simulink model "SerialSystem"  (R2014a)
settings: Solver=ode3  StartTime=0.0  StopTime=800  FixedStep=0.01  RelTol=1e-3
libraries: simulink x4
settings Model: SimulationMode=accelerator  Creator=nw010080  LastModifiedBy=nm010080
settings DebuggingCC: UnderspecifiedInitializationDetection=Classic  StateNameClashWarn=warning

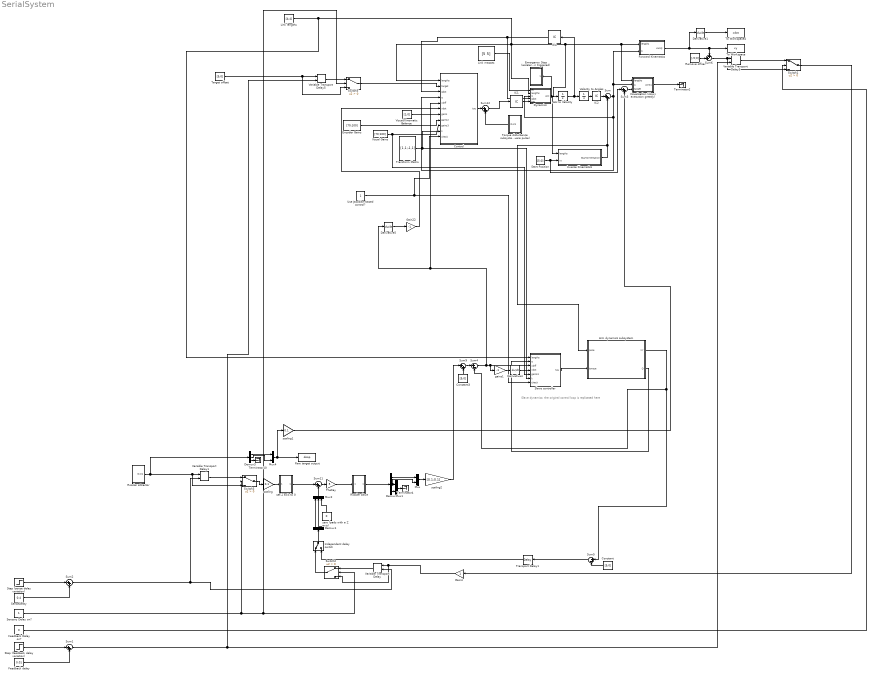
== system SerialSystem ==
  note: Slave dynamics: the original control
      | loop is replicated here
  Acc to Velocity : Integrator
  Arm dynamics subsystem : Subsystem
  Constant : Constant  Value=[5;0]
  Constant3 : Constant  Value=[5;0]
  Control : MATLAB Function  TreatAsAtomicUnit=on
  Demux : Demux  Outputs=3
  Demux1 : Demux  Outputs=2
  Demux3 : Demux  Outputs=3
  Derivative1 : Derivative
  Derivative4 : Derivative
  Derivative5 : Derivative
  Dynamics : MATLAB Function  TreatAsAtomicUnit=on
  Emergency Stop (acceleration triggered) : Subsystem
  Encoder Gains : Constant  Value=[70;100]
  Feedback Delay on? : Constant  Value=0
  Feedback delay : Constant  Value=0.01
  Forward Kinematics : MATLAB Function  TreatAsAtomicUnit=on
  Gain22 : Gain  Gain=-1
  Gain4 : Gain
  IC1 : InitialCondition  Value=[0;0]
  IC2 : InitialCondition  Value=[0;0]
  IC3 : InitialCondition  Value=[0;0]
  Independent delay switch : ManualSwitch
  Inverse Kinematics : MATLAB Function  TreatAsAtomicUnit=on
  Link lengths : Constant  Value=[4;4]
  Link masses : Constant  Value=[5 5]
  Mux : Mux  Inputs=2
  Mux1 : Mux  Inputs=2
  Mux2 : Mux  Inputs=3
  Mux4 : Mux  Inputs=2
  Raw target output : ToWorkspace  VariableName=doop  SaveFormat=Timeseries  SampleTime=-1
  Remove offset : Constant  Value=[-5;0]
  Rossler attractor : Subsystem
  Rossler slave : Subsystem
  SenseDelay : Constant  Value=0.4
  Sensory Delay on? : Constant
  Slave controller : MATLAB Function  TreatAsAtomicUnit=on
  Start Position : Constant  Value=[5;0]
  Step (feedback delay variation) : Step  Time=200  After=0.4  SampleTime=0
  Step (sense delay variation) : Step  Time=200  After=0.4  SampleTime=0
  Sum{,1..3,9,12} (6 alike) : Sum  Inputs=|++
  Sum11 : Sum  Inputs=|+-
  Sum4 : Sum  Inputs=|+-
  Sum5 : Sum  Inputs=|+-
  Sum6 : Sum  Inputs=++|
  Switch{1..3,5} (4 alike) : Switch  Criteria=u2 > Threshold
  Target offset : Constant  Value=[5;0]
  Terminator10 : Terminator
  Terminator2 : Terminator
  Terminator4 : Terminator
  TheKay : Gain  Gain=5
  To Workspace : ToWorkspace  VariableName=xy  SaveFormat=Timeseries  SampleTime=-1
  To Workspace4 : ToWorkspace  VariableName=xdot  SaveFormat=Timeseries  SampleTime=-1
  Torque disturbance subsystem (produces a single square pulse) : Subsystem
  Transform Matrix : Constant  Value=[1,1;-1,1]
  Transport Delay1 : TransportDelay  DelayTime=0.4
  Use Jacobian-based control? : Constant
  Variable Transport Delay : VariableTransportDelay  VariableDelayType=Variable transport delay  MaximumDelay=7  MaximumPoints=8024
  Variable Transport Delay1 : VariableTransportDelay  VariableDelayType=Variable transport delay  MaximumDelay=7  MaximumPoints=8024  FixedBuffer=on
  Variable Transport Delay3 : VariableTransportDelay  VariableDelayType=Variable transport delay  MaximumDelay=7  MaximumPoints=8024
  Variable Transport Delay5 : VariableTransportDelay  VariableDelayType=Variable transport delay  MaximumDelay=7  MaximumPoints=8024
  Velocity to Angles : Integrator
  Visual Gains : Constant  Value=[70;100]
  Visual/Kinematic Balance : Constant  Value=[1;0]
  Visualisation (slows execution greatly) : MATLAB Function  TreatAsAtomicUnit=on
  gains1 : Gain  Gain=-1
  scaling : Gain  Gain=0.1
  scaling1 : Gain  Gain=0.1
  scaling2 : Gain  Gain=[0.1;0.1]
  set Z axis to 0 : Subsystem
  zero (pads with a Z axis) : Constant  Value=0
  wires:
  Link lengths/1 -> Slave controller/1(lengths), Dynamics/2(lengths), Control/1(lengths), Visualisation (slows execution greatly)/1(lengths), Forward Kinematics/1(lengths), Inverse Kinematics/1(lengths)
  Visual/Kinematic Balance/1 -> Control/7(gains)
  Velocity to Angles/1 -> IC2/1
  IC2/1 -> Sum/1
  Start Position/1 -> Sum3/1, Inverse Kinematics/2(xy)
  IC3/1 -> Control/3(qdot), Dynamics/4(qdot)
  Encoder Gains/1 -> Control/8(gains2)
  Link masses/1 -> Dynamics/1(m)
  Visualisation (slows execution greatly)/1(joint1) -> Terminator2/1
  IC1/1 -> Dynamics/5(tau)
  Target offset/1 -> Switch5/3, Variable Transport Delay5/1
  Acc to Velocity/1 -> IC3/1, Velocity to Angles/1
  Derivative5/1 -> Gain22/1
  Inverse Kinematics/1(StartOrientation) -> Arm dynamics subsystem/1(pose), Sum/2
  Visual Gains/1 -> Slave controller/5(gains3), Control/9(gains3)
  gains1/1 -> Derivative4/1
  Derivative4/1 -> Slave controller/4(xdot)
  Gain22/1 -> Control/6(xdot)
  Constant3/1 -> Sum9/2
  Sum9/1 -> Sum4/1
  Sum11/1 -> TheKay/1
  Mux2/1 -> Sum11/2
  scaling/1 -> set Z axis to 0/1(In1)
  Demux/2 -> Mux/2, Mux1/1
  Demux/3 -> Mux1/2
  Mux1/1 -> Terminator4/1
  Demux/1 -> Mux/1
  zero (pads with a Z axis)/1 -> Mux2/3
  Demux1/2 -> Mux2/2
  Sum1/1 -> Variable Transport Delay5/2, Variable Transport Delay3/2
  Sum12/1 -> IC1/1
  Dynamics/1(acc) -> Acc to Velocity/1, Emergency Stop (acceleration triggered)/1(Acceleration)
  Demux1/1 -> Mux2/1
  Sum2/1 -> Variable Transport Delay/2, Variable Transport Delay1/2
  SenseDelay/1 -> Sum2/2
  Step (sense delay variation)/1 -> Sum2/1
  Sum3/1 -> Visualisation (slows execution greatly)/3(target)
  scaling2/1 -> Sum9/1
  TheKay/1 -> Rossler slave/1(In1)
  Mux/1 -> scaling2/1
  Transform Matrix/1 -> Control/10(k), Slave controller/6(k)
  Derivative1/1 -> To Workspace4/1
  set Z axis to 0/1(Out1) -> Sum11/1
  Switch5/1 -> Control/2(target)
  Feedback Delay on?/1 -> Switch1/2
  Switch3/1 -> scaling/1
  Switch1/1 -> Gain4/1
  Demux3/3 -> Terminator10/1
  Rossler slave/1(Out1) -> Demux/1
  Arm dynamics subsystem/2(Q) -> Slave controller/2(q)
  Variable Transport Delay1/1 -> Switch3/1
  Mux4/1 -> scaling1/1, Raw target output/1
  Demux3/2 -> Mux4/2
  Demux3/1 -> Mux4/1
  Sum/1 -> Control/4(q), Dynamics/3(q), Forward Kinematics/2(q), Visualisation (slows execution greatly)/2(q)
  Gain4/1 -> Variable Transport Delay/1, Switch2/3
  Remove offset/1 -> Sum6/2
  Sum6/1 -> Switch1/3, Variable Transport Delay3/1
  Slave controller/1(tau) -> Arm dynamics subsystem/2(torque)
  Arm dynamics subsystem/1(XY) -> Sum5/1, Sum4/2
  Sum4/1 -> gains1/1, Slave controller/3(xdiff), Derivative5/1, Control/5(xdiff)
  Rossler attractor/1(Out1) -> Switch3/3, Variable Transport Delay1/1, Demux3/1
  Control/1(tau) -> Sum12/1
  Variable Transport Delay3/1 -> Switch1/1
  Use Jacobian-based control?/1 -> Control/11(check), Slave controller/7(check)
  Sensory Delay on?/1 -> Switch5/2, Switch2/2, Switch3/2
  Variable Transport Delay/1 -> Switch2/1
  Variable Transport Delay5/1 -> Switch5/1
  Forward Kinematics/1(xandy) -> To Workspace/1, Sum6/1, Derivative1/1
  Sum5/1 -> Transport Delay1/1
  Constant/1 -> Sum5/2
  Transport Delay1/1 -> Independent delay switch/2
  Switch2/1 -> Independent delay switch/1
  Independent delay switch/1 -> Demux1/1
  Torque disturbance subsystem (produces a single square pulse)/1(Out1) -> Sum12/2
  Step (feedback delay variation)/1 -> Sum1/1
  Feedback delay/1 -> Sum1/2
  scaling1/1 -> Sum3/2

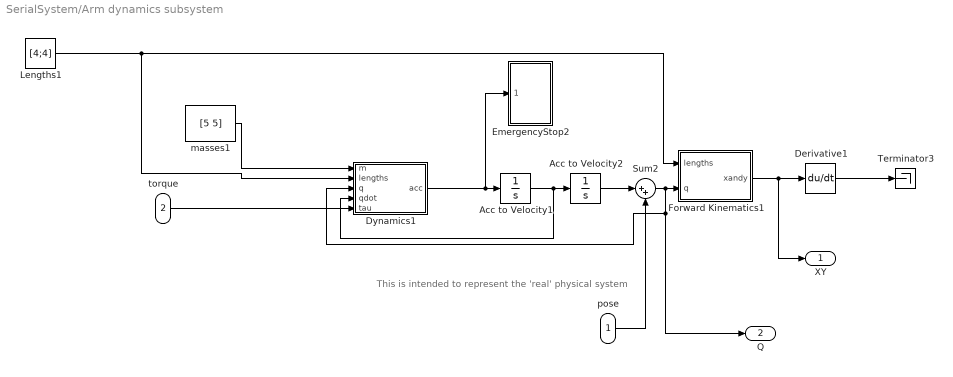
== system SerialSystem/Arm dynamics subsystem ==
  note: This is intended to represent the 'real' physical system
  pose : Inport
  torque : Inport  Port=2
  Acc to Velocity1 : Integrator
  Acc to Velocity2 : Integrator
  Derivative1 : Derivative
  Dynamics1 : MATLAB Function  TreatAsAtomicUnit=on
  EmergencyStop2 : Subsystem
  Forward Kinematics1 : MATLAB Function  TreatAsAtomicUnit=on
  Lengths1 : Constant  Value=[4;4]
  Sum2 : Sum  Inputs=|++
  Terminator3 : Terminator
  masses1 : Constant  Value=[5 5]
  XY : Outport
  Q : Outport  Port=2
  wires:
  torque/1 -> Dynamics1/5(tau)
  Forward Kinematics1/1(xandy) -> XY/1, Derivative1/1
  Acc to Velocity2/1 -> Sum2/1
  Lengths1/1 -> Dynamics1/2(lengths), Forward Kinematics1/1(lengths)
  Sum2/1 -> Q/1, Dynamics1/3(q), Forward Kinematics1/2(q)
  masses1/1 -> Dynamics1/1(m)
  Derivative1/1 -> Terminator3/1
  pose/1 -> Sum2/2
  Acc to Velocity1/1 -> Dynamics1/4(qdot), Acc to Velocity2/1
  Dynamics1/1(acc) -> EmergencyStop2/1(Acceleration), Acc to Velocity1/1

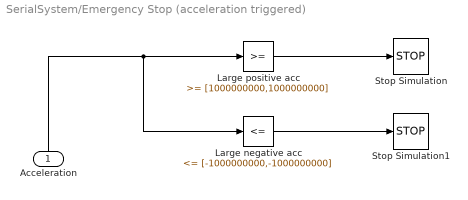
== system SerialSystem/Emergency Stop (acceleration triggered) ==
  Acceleration : Inport
  Large negative acc : simulink/Logic and Bit Operations/Compare To Constant  relop=<=  const=[-1000000000,-1000000000]  OutDataTypeStr=boolean
  Large positive acc : simulink/Logic and Bit Operations/Compare To Constant  relop=>=  const=[1000000000,1000000000]  OutDataTypeStr=boolean
  Stop Simulation : Stop
  Stop Simulation1 : Stop
  wires:
  Large negative acc/1 -> Stop Simulation1/1
  Large positive acc/1 -> Stop Simulation/1
  Acceleration/1 -> Large negative acc/1, Large positive acc/1

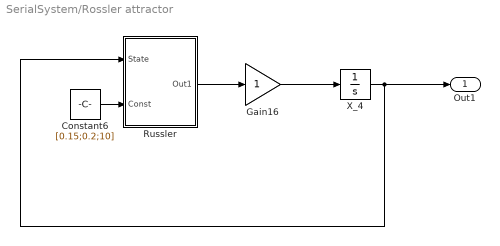
== system SerialSystem/Rossler attractor ==
  Constant6 : Constant  Value=[0.15;0.2;10]
  Gain16 : Gain
  Russler : Subsystem
  X_4 : Integrator  InitialCondition=[-1;1;0]*0
  Out1 : Outport
  wires:
  X_4/1 -> Russler/1(State), Out1/1
  Gain16/1 -> X_4/1
  Russler/1(Out1) -> Gain16/1
  Constant6/1 -> Russler/2(Const)

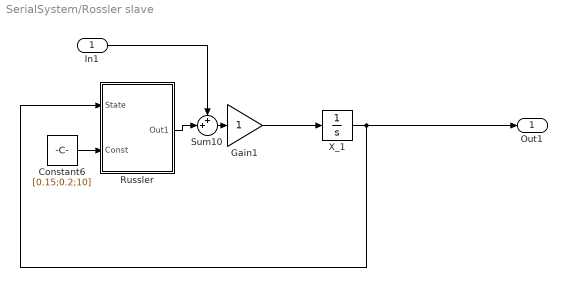
== system SerialSystem/Rossler slave ==
  In1 : Inport
  Constant6 : Constant  Value=[0.15;0.2;10]
  Gain1 : Gain
  Russler : Subsystem
  Sum10 : Sum  Inputs=++|
  X_1 : Integrator  InitialCondition=[0;0;0]
  Out1 : Outport
  wires:
  Constant6/1 -> Russler/2(Const)
  In1/1 -> Sum10/1
  Sum10/1 -> Gain1/1
  Russler/1(Out1) -> Sum10/2
  Gain1/1 -> X_1/1
  X_1/1 -> Out1/1, Russler/1(State)

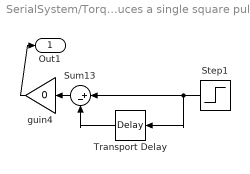
== system SerialSystem/Torque disturbance subsystem (produces a single square pulse) ==
  Step1 : Step  Time=300  SampleTime=0
  Sum13 : Sum  Inputs=|+-
  Transport Delay : TransportDelay  DelayTime=0.2
  guin4 : Gain  Gain=0
  Out1 : Outport
  wires:
  Step1/1 -> Sum13/1, Transport Delay/1
  Transport Delay/1 -> Sum13/2
  guin4/1 -> Out1/1
  Sum13/1 -> guin4/1

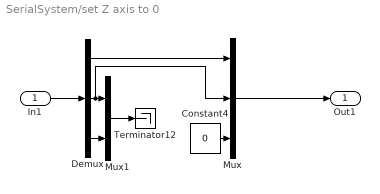
== system SerialSystem/set Z axis to 0 ==
  In1 : Inport
  Constant4 : Constant  Value=0
  Demux : Demux  Outputs=3
  Mux : Mux  Inputs=3
  Mux1 : Mux  Inputs=2
  Terminator12 : Terminator
  Out1 : Outport
  wires:
  Demux/1 -> Mux/1
  In1/1 -> Demux/1
  Mux1/1 -> Terminator12/1
  Demux/3 -> Mux1/2
  Demux/2 -> Mux/2, Mux1/1
  Constant4/1 -> Mux/3
  Mux/1 -> Out1/1

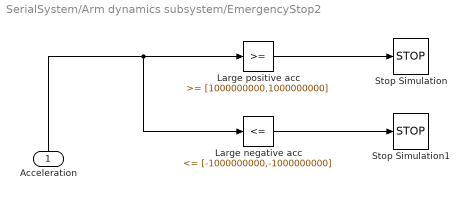
== system SerialSystem/Arm dynamics subsystem/EmergencyStop2 ==
  Acceleration : Inport
  Large negative acc : simulink/Logic and Bit Operations/Compare To Constant  relop=<=  const=[-1000000000,-1000000000]  OutDataTypeStr=boolean
  Large positive acc : simulink/Logic and Bit Operations/Compare To Constant  relop=>=  const=[1000000000,1000000000]  OutDataTypeStr=boolean
  Stop Simulation : Stop
  Stop Simulation1 : Stop
  wires:
  Large negative acc/1 -> Stop Simulation1/1
  Large positive acc/1 -> Stop Simulation/1
  Acceleration/1 -> Large negative acc/1, Large positive acc/1

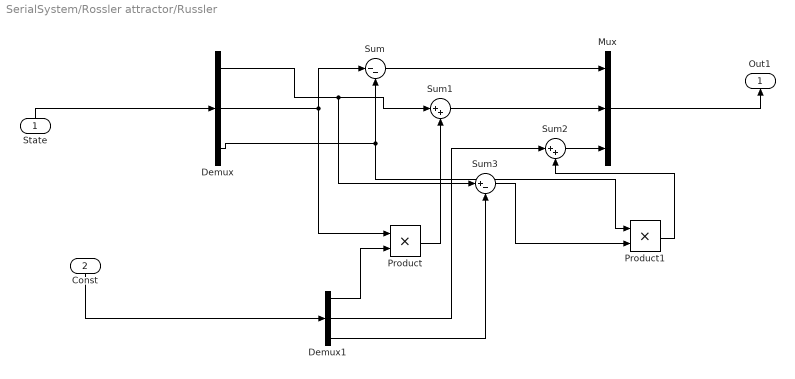
== system SerialSystem/Rossler attractor/Russler ==
  State : Inport
  Const : Inport  Port=2
  Demux : Demux  Outputs=3
  Demux1 : Demux  Outputs=3
  Mux : Mux  Inputs=3
  Product : Product
  Product1 : Product
  Sum : Sum  Inputs=|--
  Sum1 : Sum  Inputs=|++
  Sum2 : Sum  Inputs=|++
  Sum3 : Sum  Inputs=|+-
  Out1 : Outport
  wires:
  Demux1/2 -> Sum2/1
  Sum3/1 -> Product1/2
  Const/1 -> Demux1/1
  Demux/1 -> Sum3/1, Sum1/1
  Demux/2 -> Sum/1, Product/1
  Product1/1 -> Sum2/2
  Demux1/3 -> Sum3/2
  Sum/1 -> Mux/1
  Sum2/1 -> Mux/3
  Product/1 -> Sum1/2
  Mux/1 -> Out1/1
  Demux1/1 -> Product/2
  Sum1/1 -> Mux/2
  State/1 -> Demux/1
  Demux/3 -> Product1/1, Sum/2

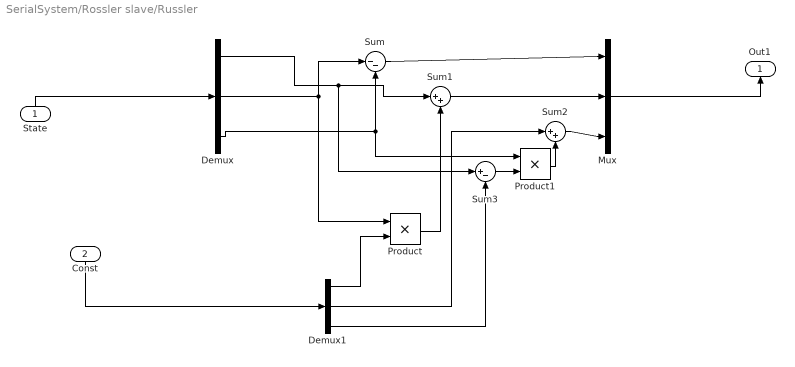
== system SerialSystem/Rossler slave/Russler ==
  State : Inport
  Const : Inport  Port=2
  Demux : Demux  Outputs=3
  Demux1 : Demux  Outputs=3
  Mux : Mux  Inputs=3
  Product : Product
  Product1 : Product
  Sum : Sum  Inputs=|--
  Sum1 : Sum  Inputs=|++
  Sum2 : Sum  Inputs=|++
  Sum3 : Sum  Inputs=|+-
  Out1 : Outport
  wires:
  Demux/3 -> Sum/2, Product1/1
  State/1 -> Demux/1
  Sum1/1 -> Mux/2
  Demux1/1 -> Product/2
  Mux/1 -> Out1/1
  Product/1 -> Sum1/2
  Sum2/1 -> Mux/3
  Sum/1 -> Mux/1
  Demux1/3 -> Sum3/2
  Product1/1 -> Sum2/2
  Demux/2 -> Product/1, Sum/1
  Demux/1 -> Sum1/1, Sum3/1
  Const/1 -> Demux1/1
  Sum3/1 -> Product1/2
  Demux1/2 -> Sum2/1

== matlab function SerialSystem/Forward Kinematics ==
  data: lengths input; xandy output; q input
function xandy  = fKinematics(lengths, q)
% forward kinematics equations
l1 = lengths(1);
l2 = lengths(2);

x = l1*cos(q(1)) + l2*cos(q(1)+q(2));
y = l1*sin(q(1)) + l2*sin(q(1)+q(2));

xandy = [x;y];

== matlab function SerialSystem/Control ==
  data: lengths input; tau output; target input; qdot input; q input; xdiff input; xdot input; gains input; gains2 input; gains3 input; k input; check input
function tau  = control(lengths, target, qdot, q, xdiff, xdot, gains,gains2, gains3, k, check)
queue = q;% get joint positions
l1 = lengths(1);
l2 = lengths(2);

if(target(1)^2 + target(2)^2 > (l1+l2-0.02)^2)% caps target to within arm reach, preventing ensuring the inverse kinematics return a real solution
    targ1 = target(1)*((l1+l2-0.02)/sqrt(target(1)^2+target(2)^2));
    targ2 = target(2)*((l1+l2-0.02)/sqrt(target(1)^2+target(2)^2));
    target = [targ1;targ2];
end

% extract gain values
m1 = gains(1);
m2 = gains(2);
kp = gains3(1);
kv = gains3(2);
gp = gains2(1);
gv = gains2(2);


% place into diagonal gain matrices
tau = [0;0];

M1 = [m1,0;0,m1];%camera gain
M2 = [m2,0;0,m2];%encoder gain

Kp = [kp,0;0,kp];% 'camera' position feedback gain
kv = [kv,0;0,kv];% 'camera' velocity feedback gain

Gp = [gp,0;0,gp];% jointspace position feedback gain
Gv = [gv,0;0,gv];% jointspace velocity feedback gain

%---------------------------------Inverse kinematics-----------------------
d1 = (target(1)^2 + target(2)^2 + l1^2 - l2^2)/(2*l1);
d2 = (target(1)^2 + target(2)^2 - l1^2 + l2^2)/(2*l2);

Q1 = atan2(target(2),target(1)) - atan2(sqrt(target(1)^2 + target(2)^2 - d1^2),d1);
Q2 = atan2(sqrt(target(1)^2 + target(2)^2 - d1^2),d1) + atan2(sqrt(target(1)^2 + target(2)^2 - d2^2),d2);
%--------------------------------------------------------------------------

desiredq = [Q1;Q2];% target joint angles

J=[-l1*sin(q(1))-l2*sin(q(1)+q(2)), -l2*sin(q(1)+q(2)); l1*cos(q(1))+l2*cos(q(1)+q(2)), l2*cos(q(1)+q(2))];% Robot arm Jacobian
if(check)
    k = J';% transpose Jacobian for force control
end

cam = M1*(Kp*k*(xdiff)-kv*k*xdot);% visual feedback terms
internal = M2*(Gp*(desiredq-queue)-Gv*qdot);%kinematic feedback terms

% true = [-l1*sin(q(1))-l2*sin(q(1)+q(2)), -l2*sin(q(1)+q(2)); l1*cos(q(1))+l2*cos(q(1)+q(2)), l2*cos(q(1)+q(2))]'*xdot;
% est = k*xdot;

tau = cam + internal;% calculate total torque

== matlab function SerialSystem/Inverse Kinematics ==
  data: lengths input; StartOrientation output; xy input
function StartOrientation  = iKinematics(lengths, xy)
l1 = lengths(1);
l2 = lengths(2);

StartOrientation = zeros(2,1);

d1 = (xy(1)^2 + xy(2)^2 + l1^2 - l2^2)/(2*l1);
d2 = (xy(1)^2 + xy(2)^2 - l1^2 + l2^2)/(2*l2);

StartOrientation(1) = atan2(xy(2),xy(1)) - atan2(sqrt(xy(1)^2 + xy(2)^2 - d1^2),d1);
StartOrientation(2) = atan2(sqrt(xy(1)^2 + xy(2)^2 - d1^2),d1) + atan2(sqrt(xy(1)^2 + xy(2)^2 - d2^2),d2);

== matlab function SerialSystem/Visualisation (slows execution greatly) ==
  data: lengths input; q input; target input; joint1 output
function joint1 = vis(lengths, q, target)
l1 = lengths(1);
l2 = lengths(2);

jointx = [0, l1*cos(q(1)), l1*cos(q(1))+l2*cos(q(1)+q(2))];% x positions of arm joints and end effector
jointy = [0, l1*sin(q(1)), l1*sin(q(1))+l2*sin(q(1)+q(2))];% y positions of arm joints and end effector

joint1 = [jointx(2);jointy(2)];

%%%%%%% Uncomment in order to see arm visualisation (slows execution) %%%%%
% coder.extrinsic('plot', 'axis', 'title');% allows MATLAB's plot function to be called
% 
% plot(jointx, jointy,'o-', target(1),target(2),'r+');% plot arm and target
% axis([0 1.5*(l1+l2) -1.5*(l1) 1.5*(l1)]);

== matlab function SerialSystem/Dynamics ==
  data: m input; lengths input; acc output; q input; qdot input; tau input
function acc  = Dyn(m, lengths, q, qdot, tau)
queue = q;
acc = [0;0];

l1 = lengths(1);% length of link one
l2 = lengths(2);% length of link two
m1 = m(1);% mass of link one
m2 = m(2);% mass of link two

lc1 = l1/2;% distance to centre of mass of link one
lc2 = l2/2;% distance to centre of mass of link two

j1 = (m1*l1^2)/3;% moment of inertia for thin, ideal pole
j2 = (m2*l2^2)/3;% placeholder

%%%%%%%%%%%%%%%%%%%%%%%%%%%% inertia matrix %%%%%%%%%%%%%%%%%%%%%%%%%%%%%%%
m11 = j1 + j2 +2*m2*l1*lc2*cos(queue(2)) + m2*l1^2 + m1*lc1^2 + m2*lc2^2;
m12 = j2 + m2*l1*lc2*cos(queue(2)) + m2*lc2^2;
m21 = m12;
m22 = j2 + m2*lc2^2;

M = [m11,m12;m21,m22];
%%%%%%%%%%%%%%%%%%%%%%%%%%%%%%%%%%%%%%%%%%%%%%%%%%%%%%%%%%%%%%%%%%%%%%%%%%%

%%%%%%%%%%%%%%%%%%%%%%%  coriolis force vector %%%%%%%%%%%%%%%%%%%%%%%%%%%%
h1 = -m2*l2*lc2*(2*qdot(1)+qdot(2))*qdot(2)*sin(queue(2));
h2 = m2*l1*lc2*qdot(1)^2*sin(queue(2));

h = [h1;h2];
%%%%%%%%%%%%%%%%%%%%%%%%%%%%%%%%%%%%%%%%%%%%%%%%%%%%%%%%%%%%%%%%%%%%%%%%%%%

acc = M\(tau-h);% solve dynamics equation for acceleration

== matlab function SerialSystem/Arm dynamics subsystem/Dynamics1 ==
  data: m input; lengths input; acc output; q input; qdot input; tau input
function acc  = Dyn(m, lengths, q, qdot, tau)
queue = q;
acc = [0;0];

l1 = lengths(1);% length of link one
l2 = lengths(2);% length of link two
m1 = m(1);% mass of link one
m2 = m(2);% mass of link two

lc1 = l1/2;% distance to centre of mass of link one
lc2 = l2/2;% distance to centre of mass of link two

j1 = (m1*l1^2)/3;% moment of inertia for thin, ideal pole
j2 = (m2*l2^2)/3;% placeholder

m11 = j1 + j2 +2*m2*l1*lc2*cos(queue(2)) + m2*l1^2 + m1*lc1^2 + m2*lc2^2;
m12 = j2 + m2*l1*lc2*cos(queue(2)) + m2*lc2^2;
m21 = m12;
m22 = j2 + m2*lc2^2;

M = [m11,m12;m21,m22];% inertia matrix


h1 = -m2*l2*lc2*(2*qdot(1)+qdot(2))*qdot(2)*sin(queue(2));% coriolis
h2 = m2*l1*lc2*qdot(1)^2*sin(queue(2));

h = [h1;h2];
acc = M\(tau-h);% solve dynamics equation for acceleration

== matlab function SerialSystem/Arm dynamics subsystem/Forward Kinematics1 ==
  data: lengths input; xandy output; q input
function xandy  = fKinematics(lengths, q)
l1 = lengths(1);
l2 = lengths(2);

x = l1*cos(q(1)) + l2*cos(q(1)+q(2));
y = l1*sin(q(1)) + l2*sin(q(1)+q(2));

xandy = [x;y];

== matlab function SerialSystem/Slave controller ==
  data: lengths input; q input; tau output; xdiff input; xdot input; gains3 input; k input; check input
function tau  = control(lengths, q, xdiff, xdot, gains3, k,  check)
queue = q;% noise added to kinematic feedback
l1 = lengths(1);
l2 = lengths(2);

kp = gains3(1);
kv = gains3(2);

%approximate transform from workspace to jointspace
tau = [0;0];



Kp = [kp,0;0,kp];% 'camera' position feedback gain
kv = [kv,0;0,kv];% 'camera' velocity feedback gain


J=[-l1*sin(q(1))-l2*sin(q(1)+q(2)), -l2*sin(q(1)+q(2)); l1*cos(q(1))+l2*cos(q(1)+q(2)), l2*cos(q(1)+q(2))];
if(check)
    k = J';
end

cam = (Kp*k*(xdiff)-kv*k*xdot);% visual feedback terms


tau = cam;% calculate total torque
